simulink model "Cooperative_Quad_Rev01_4Agents_9"  (R2017b)
settings: Solver=ode45  StartTime=0.0  StopTime=120  RelTol=1e-3  EnableMultiTasking=on
InitFcn:
  | constant_Rev01_4Agents_9
values from neighbouring files (symbols this model uses):
  alpha = 0.1    [constant_Rev01_4Agents_9.m]
  alpha1 = 0.01    [constant_Rev01_4Agents_9.m]
  AN = [     0 1 0 0 ... (first row only)    [constant_Rev01_4Agents_9.m]
  B = 1e0*eye(n)    [constant_Rev01_4Agents_9.m]
  BBT_inv = ((B'*B)^(-1))*B'    [constant_Rev01_4Agents_9.m]
  BN = [     1 0 0 0 ... (first row only)    [constant_Rev01_4Agents_9.m]
  epsilon_struct = struct('data',epsilon_InitVal)    [constant_Rev01_4Agents_9.m]
  g = 9.81    [constant_Rev01_4Agents_9.m]
  gamma_0 = 1e+1*diag([1e-3*ones(6,1);1e-0*ones(6,1)])    [constant_Rev01_4Agents_9.m]
  gamma_1 = 1e+3*diag([1e-3*ones(6,1);1e0*ones(6,1)])    [constant_Rev01_4Agents_9.m]
  H = L + BN    [constant_Rev01_4Agents_9.m]
  J = 1.2416e-3 * diag([1 1 2],0)    [constant_Rev01_4Agents_9.m]
  k1 = 1    [constant_Rev01_4Agents_9.m]
  k2 = 1    [constant_Rev01_4Agents_9.m]
  Ka = 0.01    [constant_Rev01_4Agents_9.m]
  Kd = 0.01    [constant_Rev01_4Agents_9.m]
  Kf = 1e-5    (= 1e-05)    [constant_Rev01_4Agents_9.m]
  Ki = 1    [constant_Rev01_4Agents_9.m]
  Kt = 0.01 * Kf    (= 1e-07)    [constant_Rev01_4Agents_9.m]
  Lq = 0.2    [constant_Rev01_4Agents_9.m]
  M = 2    [constant_Rev01_4Agents_9.m]
  n = 12    [constant_Rev01_4Agents_9.m]
  N = 4    [constant_Rev01_4Agents_9.m]
  n0 = 3    [constant_Rev01_4Agents_9.m]
  Observer_Gain = 100    [constant_Rev01_4Agents_9.m]
  Observer_Gain1 = 10    [constant_Rev01_4Agents_9.m]
  Q = 1e-3*eye(n)    [constant_Rev01_4Agents_9.m]
  R = 1e-0*eye(n)    [constant_Rev01_4Agents_9.m]
  rho_0 = 1e+1    (= 10)    [constant_Rev01_4Agents_9.m]
  rho_1 = 1e-1    (= 0.1)    [constant_Rev01_4Agents_9.m]
  RM_1 = RM^(-1)    [constant_Rev01_4Agents_9.m]
  T_struct = struct('data',T_InitVal)    [constant_Rev01_4Agents_9.m]
  U_dot0_M = U_dot0_m*ones(n0,1)    [constant_Rev01_4Agents_9.m]
  Upsilon_M = Upsilon_m*ones(n0,1)    [constant_Rev01_4Agents_9.m]
undefined symbols (not defined in the file or in its folder): sigbuilder_block
(part 2 of 2)

== matlab function Cooperative_Quad_Rev01_4Agents_9/Agent #3/Decenteralized Cooperaive Controller #3/Controller #3/Differentiator/Sliding differentiator1 ==
  data: Du1 output; e input; k2 parameter; alpha1 parameter
function Du1 = fcn(e,k2,alpha1)

a=k2;

ABS = abs(e);
SGN = e ./ (ABS + alpha1);
Du1 = - a*SGN;

end

== matlab function Cooperative_Quad_Rev01_4Agents_9/Agent #3/Decenteralized Cooperaive Controller #3/Controller #3/g-Estimator ==
  data: sigma input; g_hat input; P input; rho_1 parameter; gamma_1 parameter; Dg_hat output
function Dg_hat = fcn(sigma,g_hat,P,rho_1,gamma_1)

Dg_hat = - gamma_1 * P * sigma - rho_1 * gamma_1 * g_hat;

end

== matlab function Cooperative_Quad_Rev01_4Agents_9/Agent #3/Decenteralized Cooperaive Controller #3/Controller #3/g-Estimator1 ==
  data: sigma input; x input; P input; rho_0 parameter; gamma_0 parameter; Da_hat output; a_hat input
function Da_hat = fcn(sigma,x,P,rho_0,gamma_0,a_hat)

DVa_hat = - gamma_0 * P * diag(sigma) * (x - sigma) - rho_0 * gamma_0 * diag(a_hat);

Da_hat = diag(DVa_hat);

end

== matlab function Cooperative_Quad_Rev01_4Agents_9/Agent #3/Decenteralized Cooperaive Controller #3/Controller #3/main ==
  data: sigma input; zeta input; u output; Dy_d input; R parameter; P input; a_hat input; B parameter; g_hat input; x input; Q parameter; BBT_inv parameter; n parameter; Ki parameter
function u = fcn(sigma,zeta,Dy_d,R,P,a_hat,B,g_hat,x,Q,BBT_inv,n,Ki)

u1 = (1/2) * R * B' * P * sigma;
u2 = BBT_inv * (Dy_d - a_hat*x + (Ki*eye(n) + 2*(((P)^(-1)*Q)) + a_hat)*sigma - g_hat - Ki*zeta) - (3/4) * R * B' * P * sigma;

u = u1 + u2;

end

== matlab function Cooperative_Quad_Rev01_4Agents_9/Agent #3/Decenteralized Cooperaive Controller #3/Controller #3/variable change ==
  data: X input; Xd input; x_mod output; u input; xd_mod output; e_mod output; phi_d output; theta_d output
function [x_mod,xd_mod,e_mod,phi_d,theta_d] = fcn(X,Xd,u)

x_mod = X;

u0 = sqrt((u(7)^2)+(u(8)^2)+(u(9)^2));

psi_d = 0;
phi_d = asin( min(max(((sin(psi_d)*u(7) - cos(psi_d)*u(8)) / (u0+0.001)),-1),1) );
theta_d = atan( (cos(psi_d)*u(7) + sin(psi_d)*u(8)) / (u(9)+1e-3) );

PHI_d = [phi_d;theta_d;psi_d]; 

xd_mod = [Xd;PHI_d;u(1:6)];

e_mod = xd_mod - x_mod;


end

== matlab function Cooperative_Quad_Rev01_4Agents_9/Agent #3/Decenteralized Cooperaive Controller #3/Observer T#3 ==
  data: T_struct parameter; T input; DT_i output; epsilon input; epsilon_struct parameter; H parameter; BN parameter; AN parameter; T_i input; chi input; Upsilon_M parameter; epsilon_i output; N parameter; n0 parameter; Agent_Num input; Observer_Gain1 parameter; alpha parameter
function [DT_i,epsilon_i] = fcn(T_struct,T,epsilon,epsilon_struct,H,BN,AN,T_i,chi,Upsilon_M,N,n0,...
    Agent_Num,Observer_Gain1,alpha)

T_struct(1).data = T.t1;
T_struct(2).data = T.t2;
T_struct(3).data = T.t3;
T_struct(4).data = T.t4;

epsilon_struct(1).data = epsilon.eps1;
epsilon_struct(2).data = epsilon.eps2;
epsilon_struct(3).data = epsilon.eps3;
epsilon_struct(4).data = epsilon.eps4;

epsilon_i = + BN(Agent_Num,Agent_Num)*(T_i - chi);
Sum2 = zeros(N+1,n0);
for i=1:N
    epsilon_i = epsilon_i + ( AN(Agent_Num,i) * (T_i - T_struct(i).data) );  
    Sum2 = Sum2 + ( H(i,Agent_Num) * epsilon_struct(i).data );
end

Sum21 = abs(Sum2) + alpha;
SGN2 = Sum2./Sum21;

DT_i = -Observer_Gain1*epsilon_i - SGN2*diag(Upsilon_M);

end

== matlab function Cooperative_Quad_Rev01_4Agents_9/Agent #3/Decenteralized Cooperaive Controller #3/Observer q#3 ==
  data: q input; Dq_i output; tau input; H parameter; BN parameter; AN parameter; q_i input; u0 input; U_dot0_M parameter; tau_i output; N parameter; Agent_Num input; Observer_Gain parameter; n0 parameter; alpha parameter
function [Dq_i,tau_i] = fcn(q,tau,H,BN,AN,q_i,u0,U_dot0_M,N,Agent_Num,Observer_Gain,n0,alpha)

tau_i = + BN(Agent_Num,Agent_Num)*(q_i - u0);
Sum2 = zeros(n0,1);
for i=1:N
    tau_i = tau_i + ( AN(Agent_Num,i) * (q_i - q(((i-1)*n0+1):n0*i)) );  
    Sum2 = Sum2 + ( H(i,Agent_Num) * tau(((i-1)*n0+1):n0*i) );
end

Sum21 = abs(Sum2) + alpha;
SGN2 = Sum2./Sum21;

Dq_i = -Observer_Gain*tau_i - diag(SGN2)*U_dot0_M;

end

== matlab function Cooperative_Quad_Rev01_4Agents_9/Agent #3/Plant #3/MATLAB Function ==
  data: X input; u1 input; u2 input; u3 input; u4 input; t input; DX output; Kf parameter; Kt parameter; Kd parameter; Ka parameter; M parameter; J parameter; Lq parameter; g parameter
function DX = fcn(X,u1,u2,u3,u4,t,Kf,Kt,Kd,Ka,M,J,Lq,g)

F1 = Kf * u1^2;
F2 = Kf * u2^2;
F3 = Kf * u3^2;
F4 = Kf * u4^2;
 
FT = F1 + F2 + F3 + F4;

T1 = Kt * u1^2;
T2 = Kt * u2^2;
T3 = Kt * u3^2;
T4 = Kt * u4^2;

phi = X(4);
theta = X(5);
psi = X(6);

Rq = [cos(psi)*cos(theta) -sin(psi)*cos(phi)+cos(psi)*sin(theta)*sin(phi) sin(psi)*sin(phi)+cos(psi)*sin(theta)*cos(phi);
    sin(psi)*cos(theta) cos(psi)*cos(phi)+sin(psi)*sin(theta)*sin(phi) -cos(psi)*sin(phi)+sin(psi)*sin(theta)*cos(phi);
    -sin(theta) cos(theta)*sin(phi) cos(theta)*cos(phi)]; 

R_omega = [1 0 -sin(theta);
    0 cos(phi) cos(theta)*sin(phi);
    0 -sin(phi) cos(theta)*cos(phi)];

EXT_PRD = External_Product3(X(10:12),(J*X(10:12)));

DP = X(7:9);
DPHI = R_omega^(-1) * X(10:12); 
Dv = (1/M)*(Rq*[0;0;FT] - Kd*X(7:9) - M*[0;0;g]) + Rq*(1*sin(1*t))*[0;0;1];
Dw = (J^(-1))*([Lq*(F3-F1);Lq*(F4-F2);(T1-T2+T3-T4)] - Ka*X(10:12) - EXT_PRD) + (1*sin(1*t));

DX = [DP;DPHI;Dv;Dw];

end

== matlab function Cooperative_Quad_Rev01_4Agents_9/Agent #1/Decenteralized Cooperaive Controller #1/Controller #1/Differentiator/Sliding differentiator ==
  data: u output; u1 input; e input; k1 parameter; alpha1 parameter
function u = fcn(u1,e,k1,alpha1)

b=k1;

ABS = abs(e);
SGN = e ./ (ABS + alpha1);
u = u1 - b*(ABS.^0.5).*SGN;

end

== matlab function Cooperative_Quad_Rev01_4Agents_9/Agent #1/Decenteralized Cooperaive Controller #1/Controller #1/Differentiator/Sliding differentiator1 ==
  data: Du1 output; e input; k2 parameter; alpha1 parameter
function Du1 = fcn(e,k2,alpha1)

a=k2;

ABS = abs(e);
SGN = e ./ (ABS + alpha1);
Du1 = - a*SGN;

end

== matlab function Cooperative_Quad_Rev01_4Agents_9/Agent #4/Controller interpreter ==
  data: u output; U input; RM_1 parameter; n0 parameter; n parameter
function u = fcn(U,RM_1,n0,n)

y0 = sqrt((U(7)^2)+(U(8)^2)+(U(9)^2));
y1 = U(10);
y2 = U(11);
y3 = U(12);

Y = [y0;y1;y2;y3];

u = RM_1*Y;

for i=1:4
    u(i) = sqrt(abs(u(i)));
end

end

== matlab function Cooperative_Quad_Rev01_4Agents_9/Agent #4/Decenteralized Cooperaive Controller #4/Computing xd  ==
  data: q_i input; T_i input; xd output; Agent_Num input
function xd = fcn(q_i,T_i,Agent_Num)

xd = q_i + T_i(1,:)' + T_i(Agent_Num+1,:)';

end

== matlab function Cooperative_Quad_Rev01_4Agents_9/Agent #4/Decenteralized Cooperaive Controller #4/Controller #4/CARE ==
  data: P input; a_hat input; B parameter; R parameter; DP output; Q parameter
function DP = fcn(P,a_hat,B,R,Q)

DP = a_hat*P + P*a_hat' - P*B*R*B'*P + 2*Q;

end

== matlab function Cooperative_Quad_Rev01_4Agents_9/Agent #4/Decenteralized Cooperaive Controller #4/Controller #4/Differentiator/Sliding differentiator ==
  data: u output; u1 input; e input; k1 parameter; alpha1 parameter
function u = fcn(u1,e,k1,alpha1)

b=k1;

ABS = abs(e);
SGN = e ./ (ABS + alpha1);
u = u1 - b*(ABS.^0.5).*SGN;

end

== matlab function Cooperative_Quad_Rev01_4Agents_9/Agent #4/Decenteralized Cooperaive Controller #4/Controller #4/Differentiator/Sliding differentiator1 ==
  data: Du1 output; e input; k2 parameter; alpha1 parameter
function Du1 = fcn(e,k2,alpha1)

a=k2;

ABS = abs(e);
SGN = e ./ (ABS + alpha1);
Du1 = - a*SGN;

end

== matlab function Cooperative_Quad_Rev01_4Agents_9/Agent #4/Decenteralized Cooperaive Controller #4/Controller #4/g-Estimator ==
  data: sigma input; g_hat input; P input; rho_1 parameter; gamma_1 parameter; Dg_hat output
function Dg_hat = fcn(sigma,g_hat,P,rho_1,gamma_1)

Dg_hat = - gamma_1 * P * sigma - rho_1 * gamma_1 * g_hat;

end

== matlab function Cooperative_Quad_Rev01_4Agents_9/Agent #4/Decenteralized Cooperaive Controller #4/Controller #4/g-Estimator1 ==
  data: sigma input; x input; P input; rho_0 parameter; gamma_0 parameter; Da_hat output; a_hat input
function Da_hat = fcn(sigma,x,P,rho_0,gamma_0,a_hat)

DVa_hat = - gamma_0 * P * diag(sigma) * (x - sigma) - rho_0 * gamma_0 * diag(a_hat);

Da_hat = diag(DVa_hat);

end

== matlab function Cooperative_Quad_Rev01_4Agents_9/Agent #4/Decenteralized Cooperaive Controller #4/Controller #4/main ==
  data: sigma input; zeta input; u output; Dy_d input; R parameter; P input; a_hat input; B parameter; g_hat input; x input; Q parameter; BBT_inv parameter; n parameter; Ki parameter
function u = fcn(sigma,zeta,Dy_d,R,P,a_hat,B,g_hat,x,Q,BBT_inv,n,Ki)

u1 = (1/2) * R * B' * P * sigma;
u2 = BBT_inv * (Dy_d - a_hat*x + (Ki*eye(n) + 2*(((P)^(-1)*Q)) + a_hat)*sigma - g_hat - Ki*zeta) - (3/4) * R * B' * P * sigma;

u = u1 + u2;

end

== matlab function Cooperative_Quad_Rev01_4Agents_9/Agent #4/Decenteralized Cooperaive Controller #4/Controller #4/variable change ==
  data: X input; Xd input; x_mod output; u input; xd_mod output; e_mod output; phi_d output; theta_d output
function [x_mod,xd_mod,e_mod,phi_d,theta_d] = fcn(X,Xd,u)

x_mod = X;

u0 = sqrt((u(7)^2)+(u(8)^2)+(u(9)^2));

psi_d = 0;
phi_d = asin( min(max(((sin(psi_d)*u(7) - cos(psi_d)*u(8)) / (u0+0.001)),-1),1) );
theta_d = atan( (cos(psi_d)*u(7) + sin(psi_d)*u(8)) / (u(9)+1e-3) );

PHI_d = [phi_d;theta_d;psi_d]; 

xd_mod = [Xd;PHI_d;u(1:6)];

e_mod = xd_mod - x_mod;


end

== matlab function Cooperative_Quad_Rev01_4Agents_9/Agent #4/Decenteralized Cooperaive Controller #4/Observer T#4 ==
  data: T_struct parameter; T input; DT_i output; epsilon input; epsilon_struct parameter; H parameter; BN parameter; AN parameter; T_i input; chi input; Upsilon_M parameter; epsilon_i output; N parameter; n0 parameter; Agent_Num input; Observer_Gain1 parameter; alpha parameter
function [DT_i,epsilon_i] = fcn(T_struct,T,epsilon,epsilon_struct,H,BN,AN,T_i,chi,Upsilon_M,N,n0,...
    Agent_Num,Observer_Gain1,alpha)

T_struct(1).data = T.t1;
T_struct(2).data = T.t2;
T_struct(3).data = T.t3;
T_struct(4).data = T.t4;

epsilon_struct(1).data = epsilon.eps1;
epsilon_struct(2).data = epsilon.eps2;
epsilon_struct(3).data = epsilon.eps3;
epsilon_struct(4).data = epsilon.eps4;

epsilon_i = + BN(Agent_Num,Agent_Num)*(T_i - chi);
Sum2 = zeros(N+1,n0);
for i=1:N
    epsilon_i = epsilon_i + ( AN(Agent_Num,i) * (T_i - T_struct(i).data) );  
    Sum2 = Sum2 + ( H(i,Agent_Num) * epsilon_struct(i).data );
end

Sum21 = abs(Sum2) + alpha;
SGN2 = Sum2./Sum21;

DT_i = -Observer_Gain1*epsilon_i - SGN2*diag(Upsilon_M);

end

== matlab function Cooperative_Quad_Rev01_4Agents_9/Agent #4/Decenteralized Cooperaive Controller #4/Observer q#4 ==
  data: q input; Dq_i output; tau input; H parameter; BN parameter; AN parameter; q_i input; u0 input; U_dot0_M parameter; tau_i output; N parameter; Agent_Num input; Observer_Gain parameter; n0 parameter; alpha parameter
function [Dq_i,tau_i] = fcn(q,tau,H,BN,AN,q_i,u0,U_dot0_M,N,Agent_Num,Observer_Gain,n0,alpha)

tau_i = + BN(Agent_Num,Agent_Num)*(q_i - u0);
Sum2 = zeros(n0,1);
for i=1:N
    tau_i = tau_i + ( AN(Agent_Num,i) * (q_i - q(((i-1)*n0+1):n0*i)) );  
    Sum2 = Sum2 + ( H(i,Agent_Num) * tau(((i-1)*n0+1):n0*i) );
end

Sum21 = abs(Sum2) + alpha;
SGN2 = Sum2./Sum21;

Dq_i = -Observer_Gain*tau_i - diag(SGN2)*U_dot0_M;

end

== matlab function Cooperative_Quad_Rev01_4Agents_9/Agent #4/Plant #4/MATLAB Function ==
  data: X input; u1 input; u2 input; u3 input; u4 input; t input; DX output; Kf parameter; Kt parameter; Kd parameter; Ka parameter; M parameter; J parameter; Lq parameter; g parameter
function DX = fcn(X,u1,u2,u3,u4,t,Kf,Kt,Kd,Ka,M,J,Lq,g)

F1 = Kf * u1^2;
F2 = Kf * u2^2;
F3 = Kf * u3^2;
F4 = Kf * u4^2;
 
FT = F1 + F2 + F3 + F4;

T1 = Kt * u1^2;
T2 = Kt * u2^2;
T3 = Kt * u3^2;
T4 = Kt * u4^2;

phi = X(4);
theta = X(5);
psi = X(6);

Rq = [cos(psi)*cos(theta) -sin(psi)*cos(phi)+cos(psi)*sin(theta)*sin(phi) sin(psi)*sin(phi)+cos(psi)*sin(theta)*cos(phi);
    sin(psi)*cos(theta) cos(psi)*cos(phi)+sin(psi)*sin(theta)*sin(phi) -cos(psi)*sin(phi)+sin(psi)*sin(theta)*cos(phi);
    -sin(theta) cos(theta)*sin(phi) cos(theta)*cos(phi)]; 

R_omega = [1 0 -sin(theta);
    0 cos(phi) cos(theta)*sin(phi);
    0 -sin(phi) cos(theta)*cos(phi)];

EXT_PRD = External_Product3(X(10:12),(J*X(10:12)));

DP = X(7:9);
DPHI = R_omega^(-1) * X(10:12); 
Dv = (1/M)*(Rq*[0;0;FT] - Kd*X(7:9) - M*[0;0;g]) + Rq*(1*sin(1*t))*[0;0;1];
Dw = (J^(-1))*([Lq*(F3-F1);Lq*(F4-F2);(T1-T2+T3-T4)] - Ka*X(10:12) - EXT_PRD) + (1*sin(1*t));

DX = [DP;DPHI;Dv;Dw];

end

== matlab function Cooperative_Quad_Rev01_4Agents_9/Data Bus /Reference Trajectory/formation ==
  data: r_form_x input; chi output; r_form_y input; r_form_z input
function chi = fcn(r_form_x,r_form_y,r_form_z)

Delta_form = [...
    +r_form_x +r_form_y +r_form_z;
    -r_form_x +r_form_y -r_form_z;
    -r_form_x -r_form_y +2*r_form_z;
    +r_form_x -r_form_y -2*r_form_z];

chi = [0 0 0;
    Delta_form];

end

== matlab function Cooperative_Quad_Rev01_4Agents_9/Data Bus /For matrix Plot1/MATLAB Function ==
  data: u input; y output
function y = fcn(u)
S1 = size(u,1);
S2 = size(u,2);

y = zeros(S1*S2,1);
num = 0;
for i=1:S1
    for j=1:S2
        num = num + 1;
        y(num,1) = u(i,j);
    end
end

end

== matlab function Cooperative_Quad_Rev01_4Agents_9/Data Bus /For matrix Plot2/MATLAB Function ==
  data: u input; y output
function y = fcn(u)
S1 = size(u,1);
S2 = size(u,2);

y = zeros(S1*S2,1);
num = 0;
for i=1:S1
    for j=1:S2
        num = num + 1;
        y(num,1) = u(i,j);
    end
end

end

== matlab function Cooperative_Quad_Rev01_4Agents_9/Data Bus /For matrix Plot3/MATLAB Function ==
  data: u input; y output
function y = fcn(u)
S1 = size(u,1);
S2 = size(u,2);

y = zeros(S1*S2,1);
num = 0;
for i=1:S1
    for j=1:S2
        num = num + 1;
        y(num,1) = u(i,j);
    end
end

end

== matlab function Cooperative_Quad_Rev01_4Agents_9/Data Bus /For matrix Plot4/MATLAB Function ==
  data: u input; y output
function y = fcn(u)
S1 = size(u,1);
S2 = size(u,2);

y = zeros(S1*S2,1);
num = 0;
for i=1:S1
    for j=1:S2
        num = num + 1;
        y(num,1) = u(i,j);
    end
end

end

== matlab function Cooperative_Quad_Rev01_4Agents_9/Data Bus /For matrix Plot5/MATLAB Function ==
  data: u input; y output
function y = fcn(u)
S1 = size(u,1);
S2 = size(u,2);

y = zeros(S1*S2,1);
num = 0;
for i=1:S1
    for j=1:S2
        num = num + 1;
        y(num,1) = u(i,j);
    end
end

end

== matlab function Cooperative_Quad_Rev01_4Agents_9/Data Bus /For matrix Plot6/MATLAB Function ==
  data: u input; y output
function y = fcn(u)
S1 = size(u,1);
S2 = size(u,2);

y = zeros(S1*S2,1);
num = 0;
for i=1:S1
    for j=1:S2
        num = num + 1;
        y(num,1) = u(i,j);
    end
end

end

== matlab function Cooperative_Quad_Rev01_4Agents_9/Data Bus /For matrix Plot7/MATLAB Function ==
  data: u input; y output
function y = fcn(u)
S1 = size(u,1);
S2 = size(u,2);

y = zeros(S1*S2,1);
num = 0;
for i=1:S1
    for j=1:S2
        num = num + 1;
        y(num,1) = u(i,j);
    end
end

end

== matlab function Cooperative_Quad_Rev01_4Agents_9/Data Bus /For matrix Plot8/MATLAB Function ==
  data: u input; y output
function y = fcn(u)
S1 = size(u,1);
S2 = size(u,2);

y = zeros(S1*S2,1);
num = 0;
for i=1:S1
    for j=1:S2
        num = num + 1;
        y(num,1) = u(i,j);
    end
end

end

== matlab function Cooperative_Quad_Rev01_4Agents_9/Data Bus /For matrix Plot9/MATLAB Function ==
  data: u input; y output
function y = fcn(u)
S1 = size(u,1);
S2 = size(u,2);

y = zeros(S1*S2,1);
num = 0;
for i=1:S1
    for j=1:S2
        num = num + 1;
        y(num,1) = u(i,j);
    end
end

end

== matlab function Cooperative_Quad_Rev01_4Agents_9/Data Bus /For matrix Plot/MATLAB Function ==
  data: u input; y output
function y = fcn(u)
S1 = size(u,1);
S2 = size(u,2);

y = zeros(S1*S2,1);
num = 0;
for i=1:S1
    for j=1:S2
        num = num + 1;
        y(num,1) = u(i,j);
    end
end

end

== matlab function Cooperative_Quad_Rev01_4Agents_9/Data Bus /For matrix Plot10/MATLAB Function ==
  data: u input; y output
function y = fcn(u)
S1 = size(u,1);
S2 = size(u,2);

y = zeros(S1*S2,1);
num = 0;
for i=1:S1
    for j=1:S2
        num = num + 1;
        y(num,1) = u(i,j);
    end
end

end

== matlab function Cooperative_Quad_Rev01_4Agents_9/Data Bus /For matrix Plot11/MATLAB Function ==
  data: u input; y output
function y = fcn(u)
S1 = size(u,1);
S2 = size(u,2);

y = zeros(S1*S2,1);
num = 0;
for i=1:S1
    for j=1:S2
        num = num + 1;
        y(num,1) = u(i,j);
    end
end

end

== matlab function Cooperative_Quad_Rev01_4Agents_9/Data Bus /For matrix Plot12/MATLAB Function ==
  data: u input; y output
function y = fcn(u)
S1 = size(u,1);
S2 = size(u,2);

y = zeros(S1*S2,1);
num = 0;
for i=1:S1
    for j=1:S2
        num = num + 1;
        y(num,1) = u(i,j);
    end
end

end

== matlab function Cooperative_Quad_Rev01_4Agents_9/Data Bus /For matrix Plot13/MATLAB Function ==
  data: u input; y output
function y = fcn(u)
S1 = size(u,1);
S2 = size(u,2);

y = zeros(S1*S2,1);
num = 0;
for i=1:S1
    for j=1:S2
        num = num + 1;
        y(num,1) = u(i,j);
    end
end

end

== matlab function Cooperative_Quad_Rev01_4Agents_9/Data Bus /For matrix Plot14/MATLAB Function ==
  data: u input; y output
function y = fcn(u)
S1 = size(u,1);
S2 = size(u,2);

y = zeros(S1*S2,1);
num = 0;
for i=1:S1
    for j=1:S2
        num = num + 1;
        y(num,1) = u(i,j);
    end
end

end

== matlab function Cooperative_Quad_Rev01_4Agents_9/Data Bus /For matrix Plot15/MATLAB Function ==
  data: u input; y output
function y = fcn(u)
S1 = size(u,1);
S2 = size(u,2);

y = zeros(S1*S2,1);
num = 0;
for i=1:S1
    for j=1:S2
        num = num + 1;
        y(num,1) = u(i,j);
    end
end

end

== matlab function Cooperative_Quad_Rev01_4Agents_9/Agent #1/Decenteralized Cooperaive Controller #1/Controller #1/CARE ==
  data: P input; a_hat input; B parameter; R parameter; DP output; Q parameter
function DP = fcn(P,a_hat,B,R,Q)

DP = a_hat*P + P*a_hat' - P*B*R*B'*P + 2*Q;

end

== matlab function Cooperative_Quad_Rev01_4Agents_9/Agent #1/Decenteralized Cooperaive Controller #1/Controller #1/g-Estimator ==
  data: sigma input; g_hat input; P input; rho_1 parameter; gamma_1 parameter; Dg_hat output
function Dg_hat = fcn(sigma,g_hat,P,rho_1,gamma_1)

Dg_hat = - gamma_1 * P * sigma - rho_1 * gamma_1 * g_hat;

end

== matlab function Cooperative_Quad_Rev01_4Agents_9/Agent #1/Decenteralized Cooperaive Controller #1/Controller #1/A-Estimator ==
  data: sigma input; x input; P input; rho_0 parameter; gamma_0 parameter; Da_hat output; a_hat input
function Da_hat = fcn(sigma,x,P,rho_0,gamma_0,a_hat)

DVa_hat = - gamma_0 * P * diag(sigma) * (x - sigma) - rho_0 * gamma_0 * diag(a_hat);

Da_hat = diag(DVa_hat);

end

== matlab function Cooperative_Quad_Rev01_4Agents_9/Agent #1/Decenteralized Cooperaive Controller #1/Controller #1/main ==
  data: sigma input; zeta input; u output; Dy_d input; R parameter; P input; a_hat input; B parameter; g_hat input; x input; Q parameter; BBT_inv parameter; n parameter; Ki parameter
function u = fcn(sigma,zeta,Dy_d,R,P,a_hat,B,g_hat,x,Q,BBT_inv,n,Ki)

u1 = (1/2) * R * B' * P * sigma;
u2 = BBT_inv * (Dy_d - a_hat*x + (Ki*eye(n) + 2*(((P)^(-1)*Q)) + a_hat)*sigma - g_hat - Ki*zeta) - (3/4) * R * B' * P * sigma;

u = u1 + u2;

end

== matlab function Cooperative_Quad_Rev01_4Agents_9/Agent #1/Decenteralized Cooperaive Controller #1/Controller #1/variable change ==
  data: X input; Xd input; x_mod output; u input; xd_mod output; e_mod output; phi_d output; theta_d output
function [x_mod,xd_mod,e_mod,phi_d,theta_d] = fcn(X,Xd,u)

x_mod = X;

u0 = sqrt((u(7)^2)+(u(8)^2)+(u(9)^2));

psi_d = 0;
phi_d = asin( min(max(((sin(psi_d)*u(7) - cos(psi_d)*u(8)) / (u0+0.001)),-1),1) );
theta_d = atan( (cos(psi_d)*u(7) + sin(psi_d)*u(8)) / (u(9)+1e-3) );

PHI_d = [phi_d;theta_d;psi_d]; 

xd_mod = [Xd;PHI_d;u(1:6)];

e_mod = xd_mod - x_mod;


end
